simulink model "RTForwardVehicleSensorFusionTarget"  (R2024b)
settings: Solver=FixedStepAuto  StartTime=0.0  StopTime=Inf  RelTol=1e-3
PostLoadFcn:
  | helperSLForwardVehicleSensorFusionTargetSetup
undefined symbols (not defined in the file or in its folder): maxNumRadarDets, maxNumTracks, maxNumVisionDets, Ts
libraries: slrealtimeiplib x3, slrealtimeutilitieslib x3, simulink x2
CloseFcn:
  | helperSLForwardVehicleSensorFusionTargetCleanUp
settings Model: SimulationMode=external  Creator=The MathWorks, Inc.  LastModifiedBy=The MathWorks, Inc.
settings SolverCC: ConcurrentTasks=on  PositivePriorityOrder=on  MaxZcPerStep=1
settings DataIOCC: SignalLoggingName=rt_logsout
settings OptimizationCC: BlockReduction=off  OptimizeBlockIOStorage=off
settings DebuggingCC: TasksWithSamePriorityMsg=none  UnconnectedInputMsg=warning  UnconnectedOutputMsg=warning  UnconnectedLineMsg=warning  SubsystemReferenceDiagnosticForUnitTest=warning
settings HardwareCC: ProdBitPerLong=64  ProdLongLongMode=on  ProdHWDeviceType=Intel->x86-64 (Linux 64)
settings ModelReferenceCC: EnableRefExpFcnMdlSchedulingChecks=on
settings SFSimCC: SimTargetLang=C++
settings RTWCC: Description=Simulink Real-Time  SystemTargetFile=slrealtime.tlc  TemplateMakefile=slrealtime_default_tmf  Toolchain=Simulink Real-Time Toolchain  BuildConfiguration=Faster Runs  CodeExecutionProfiling=on  TargetLang=C++  GPUComputeCapability=3.5  DLArmComputeVersion=19.05
settings CodeAppCC: MaxIdLength=256
settings SimulinkRealTimeTargetCC: InstructionSetFMA=off  LogToMDFFile=off

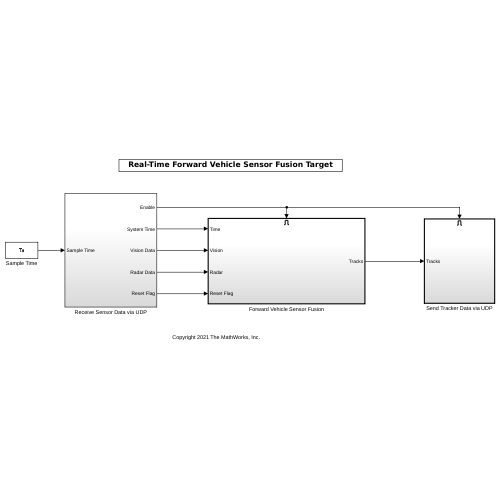
[thumbnail: Simulink's stored preview of the top-level diagram]
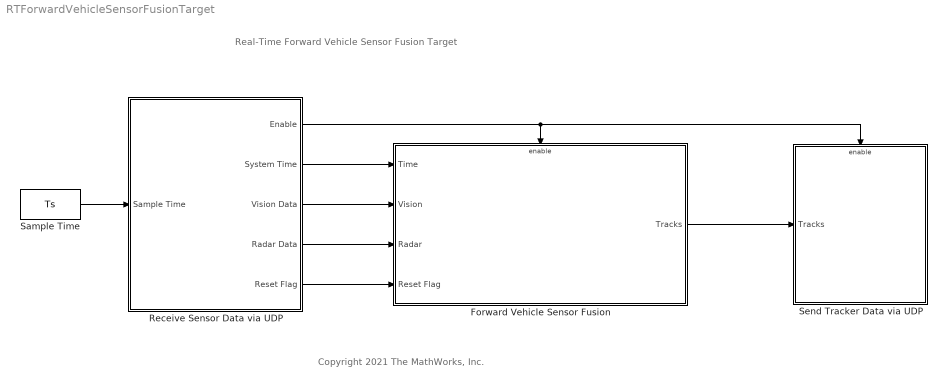
== system RTForwardVehicleSensorFusionTarget ==
  note: Real-Time Forward Vehicle Sensor Fusion Target
  note: Copyright 2021 The MathWorks, Inc.
  Forward Vehicle Sensor Fusion : Subsystem
  Receive Sensor Data via UDP : Subsystem
  Sample Time : Constant  Value=Ts  SampleTime=Ts
  Send Tracker Data via UDP : Subsystem
  wires:
  Sample Time/1 -> Receive Sensor Data via UDP/1(Sample Time)
  Receive Sensor Data via UDP/2(System Time) -> Forward Vehicle Sensor Fusion/1(Time)
  Receive Sensor Data via UDP/3(Vision Data) -> Forward Vehicle Sensor Fusion/2(Vision)
  Receive Sensor Data via UDP/4(Radar Data) -> Forward Vehicle Sensor Fusion/3(Radar)
  Receive Sensor Data via UDP/1(Enable) -> Forward Vehicle Sensor Fusion/Enable, Send Tracker Data via UDP/Enable
  Forward Vehicle Sensor Fusion/1(Tracks) -> Send Tracker Data via UDP/1(Tracks)
  Receive Sensor Data via UDP/5(Reset Flag) -> Forward Vehicle Sensor Fusion/4(Reset Flag)

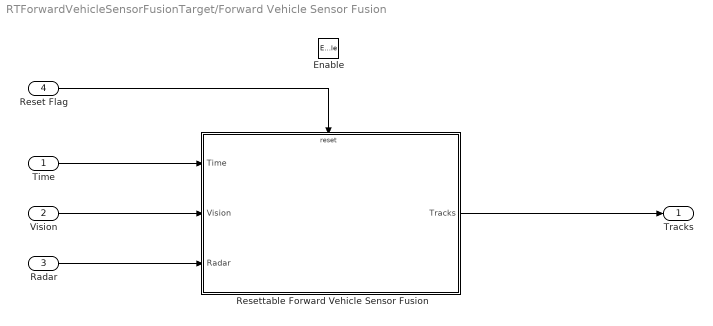
== system RTForwardVehicleSensorFusionTarget/Forward Vehicle Sensor Fusion ==
  Time : Inport
  Vision : Inport  Port=2  OutDataTypeStr=Bus: BusVision
  Radar : Inport  Port=3  OutDataTypeStr=Bus: BusRadar
  Reset Flag : Inport  Port=4
  Enable : EnablePort
  Resettable Forward Vehicle Sensor Fusion : Subsystem  TreatAsAtomicUnit=on
  Tracks : Outport
  wires:
  Time/1 -> Resettable Forward Vehicle Sensor Fusion/1(Time)
  Vision/1 -> Resettable Forward Vehicle Sensor Fusion/2(Vision)
  Radar/1 -> Resettable Forward Vehicle Sensor Fusion/3(Radar)
  Resettable Forward Vehicle Sensor Fusion/1(Tracks) -> Tracks/1
  Reset Flag/1 -> Resettable Forward Vehicle Sensor Fusion/Reset

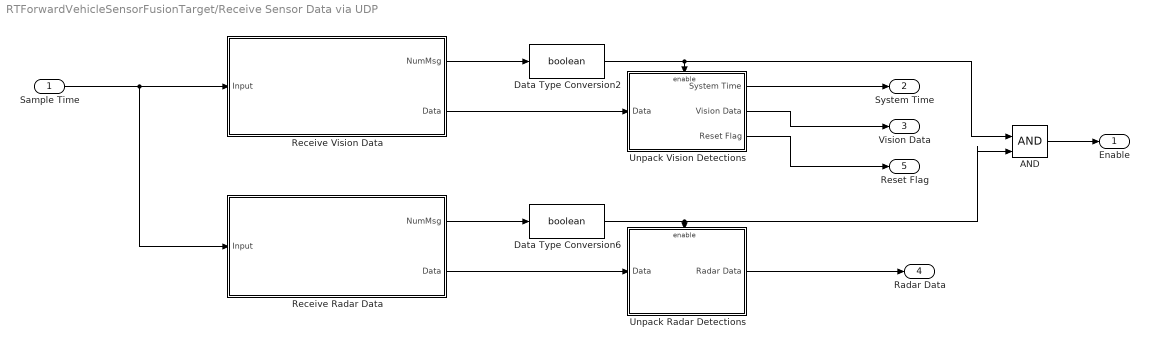
== system RTForwardVehicleSensorFusionTarget/Receive Sensor Data via UDP ==
  Sample Time : Inport
  AND : Logic  IconShape=distinctive  AllPortsSameDT=off  OutDataTypeStr=boolean
  Data Type Conversion2 : DataTypeConversion  OutDataTypeStr=boolean  SaturateOnIntegerOverflow=off  RndMeth=Floor
  Data Type Conversion6 : DataTypeConversion  OutDataTypeStr=boolean  SaturateOnIntegerOverflow=off  RndMeth=Floor
  Receive Radar Data : Subsystem
  Receive Vision Data : Subsystem
  Unpack Radar Detections : Subsystem
  Unpack Vision Detections : Subsystem
  Enable : Outport
  System Time : Outport  Port=2
  Vision Data : Outport  Port=3  OutDataTypeStr=Bus: BusVision
  Radar Data : Outport  Port=4  OutDataTypeStr=Bus: BusRadar
  Reset Flag : Outport  Port=5
  wires:
  Receive Vision Data/1(NumMsg) -> Data Type Conversion2/1
  Data Type Conversion2/1 -> AND/1, Unpack Vision Detections/Enable
  Receive Vision Data/2(Data) -> Unpack Vision Detections/1(Data)
  Unpack Vision Detections/1(System Time) -> System Time/1
  Unpack Radar Detections/1(Radar Data) -> Radar Data/1
  Receive Radar Data/2(Data) -> Unpack Radar Detections/1(Data)
  Receive Radar Data/1(NumMsg) -> Data Type Conversion6/1
  Data Type Conversion6/1 -> Unpack Radar Detections/Enable, AND/2
  Sample Time/1 -> Receive Radar Data/1(Input), Receive Vision Data/1(Input)
  Unpack Vision Detections/2(Vision Data) -> Vision Data/1
  AND/1 -> Enable/1
  Unpack Vision Detections/3(Reset Flag) -> Reset Flag/1

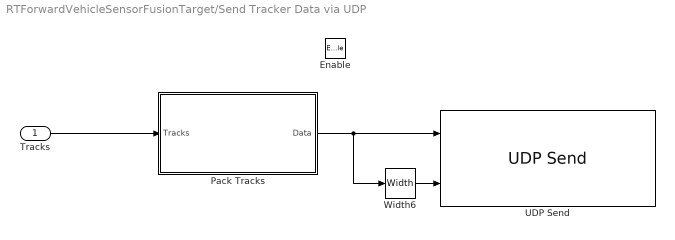
== system RTForwardVehicleSensorFusionTarget/Send Tracker Data via UDP ==
  Tracks : Inport
  Enable : EnablePort
  Pack Tracks : Subsystem
  UDP Send : slrealtimeiplib/UDP Send  useHostTargetConn=on  toAddress=10.1.10.16  toPort=8021  sampleTime=-1  enableMessage=off  ipAddress=10.1.10.17  localPort=-1
  Width6 : Width
  wires:
  Pack Tracks/1(Data) -> Width6/1, UDP Send/1
  Width6/1 -> UDP Send/2
  Tracks/1 -> Pack Tracks/1(Tracks)

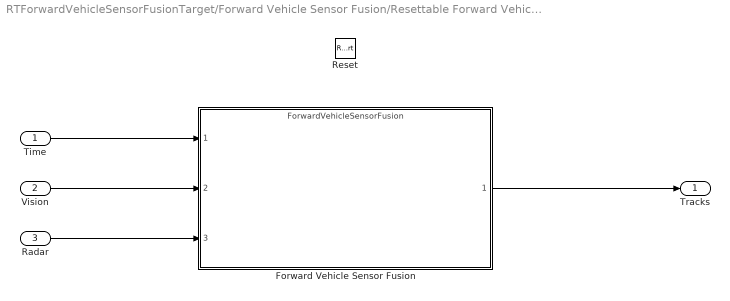
== system RTForwardVehicleSensorFusionTarget/Forward Vehicle Sensor Fusion/Resettable Forward Vehicle Sensor Fusion ==
  Time : Inport
  Vision : Inport  Port=2  OutDataTypeStr=Bus: BusVision
  Radar : Inport  Port=3  OutDataTypeStr=Bus: BusRadar
  Reset : ResetPort  DisableCoverage=on
  Forward Vehicle Sensor Fusion : ModelReference  ModelNameDialog=ForwardVehicleSensorFusion.slx  SimulationMode=Normal  CodeInterface=Top model  ModelReferenceVersion=10.0
  Tracks : Outport
  wires:
  Forward Vehicle Sensor Fusion/1 -> Tracks/1
  Time/1 -> Forward Vehicle Sensor Fusion/1
  Vision/1 -> Forward Vehicle Sensor Fusion/2
  Radar/1 -> Forward Vehicle Sensor Fusion/3

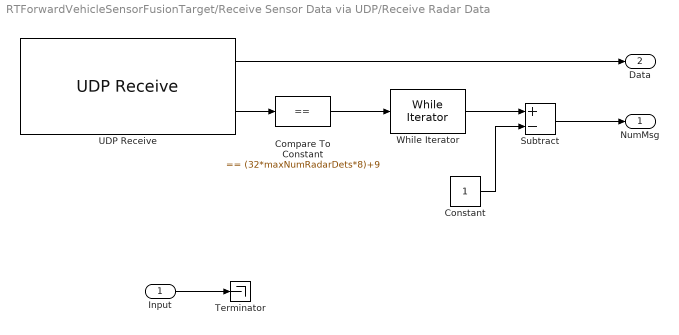
== system RTForwardVehicleSensorFusionTarget/Receive Sensor Data via UDP/Receive Radar Data ==
  Input : Inport
  Compare To Constant : simulink/Logic and Bit Operations/Compare To Constant  relop===  const=(32*maxNumRadarDets*8)+9  OutDataTypeStr=boolean
  Constant : Constant
  Subtract : Sum  Inputs=+-
  Terminator : Terminator
  UDP Receive : slrealtimeiplib/UDP Receive  useHostTargetConn=on  ipAddress=10.1.10.17  localPort=8002  rcvWidth=(32*maxNumRadarDets*8)+9  rcvFmAny=off  fmAddress=10.1.10.16  sampleTime=-1  enableMessage=off  maxPackets=1
  While Iterator : WhileIterator  WhileBlockType=do-while  ResetStates=reset  ShowIterationPort=on
  NumMsg : Outport
  Data : Outport  Port=2
  wires:
  Input/1 -> Terminator/1
  UDP Receive/2 -> Compare To Constant/1
  Subtract/1 -> NumMsg/1
  UDP Receive/1 -> Data/1
  Compare To Constant/1 -> While Iterator/1
  Constant/1 -> Subtract/2
  While Iterator/1 -> Subtract/1

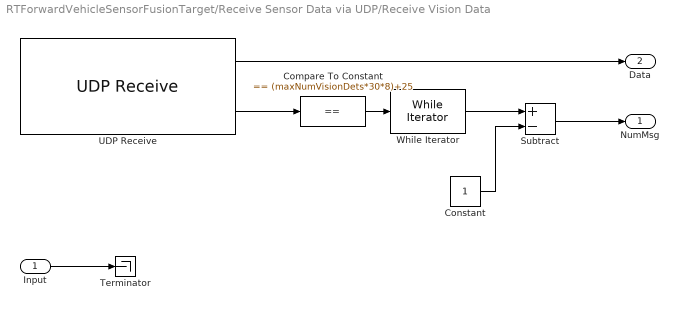
== system RTForwardVehicleSensorFusionTarget/Receive Sensor Data via UDP/Receive Vision Data ==
  Input : Inport
  Compare To Constant : simulink/Logic and Bit Operations/Compare To Constant  relop===  const=(maxNumVisionDets*30*8)+25  OutDataTypeStr=boolean
  Constant : Constant
  Subtract : Sum  Inputs=+-
  Terminator : Terminator
  UDP Receive : slrealtimeiplib/UDP Receive  useHostTargetConn=on  ipAddress=10.1.10.17  localPort=8001  rcvWidth=(maxNumVisionDets*30*8)+25  rcvFmAny=off  fmAddress=10.1.10.16  sampleTime=-1  enableMessage=off  maxPackets=1
  While Iterator : WhileIterator  WhileBlockType=do-while  ResetStates=reset  ShowIterationPort=on
  NumMsg : Outport
  Data : Outport  Port=2
  wires:
  Input/1 -> Terminator/1
  Compare To Constant/1 -> While Iterator/1
  UDP Receive/1 -> Data/1
  Constant/1 -> Subtract/2
  Subtract/1 -> NumMsg/1
  UDP Receive/2 -> Compare To Constant/1
  While Iterator/1 -> Subtract/1

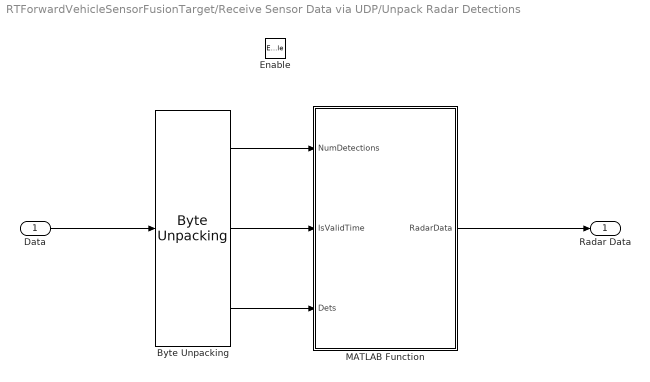
== system RTForwardVehicleSensorFusionTarget/Receive Sensor Data via UDP/Unpack Radar Detections ==
  Data : Inport
  Enable : EnablePort
  "Byte Unpacking " : slrealtimeutilitieslib/Byte Unpacking  MaskUnpackedDataTypes={'double', 'boolean', ['double']}  MaskUnpackedDataSizes={1,1,32*maxNumRadarDets}  MaskAlignment=1
  MATLAB Function : MATLAB Function  TreatAsAtomicUnit=on  mask{structObj=Simulink.Bus.createMATLABStruct('BusRadar');, maxNumDets=maxNumRadarDets}
      mask prompts: structObj "Output struct"
  Radar Data : Outport
  wires:
  "Byte Unpacking "/3 -> MATLAB Function/3(Dets)
  "Byte Unpacking "/2 -> MATLAB Function/2(IsValidTime)
  "Byte Unpacking "/1 -> MATLAB Function/1(NumDetections)
  Data/1 -> "Byte Unpacking "/1
  MATLAB Function/1(RadarData) -> Radar Data/1

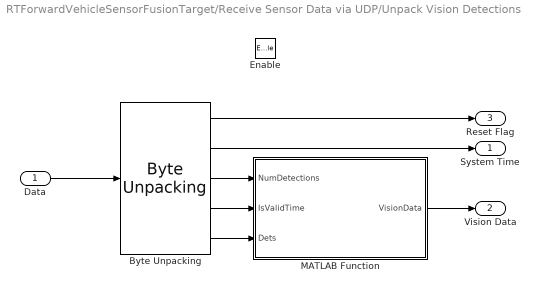
== system RTForwardVehicleSensorFusionTarget/Receive Sensor Data via UDP/Unpack Vision Detections ==
  Data : Inport
  Enable : EnablePort
  "Byte Unpacking " : slrealtimeutilitieslib/Byte Unpacking  MaskUnpackedDataTypes={'double','double','double', 'boolean', ['double']}  MaskUnpackedDataSizes={1,1,1,1,30*maxNumVisionDets}  MaskAlignment=1
  MATLAB Function : MATLAB Function  TreatAsAtomicUnit=on  mask{structObj=Simulink.Bus.createMATLABStruct('BusVision');, maxNumDets=maxNumVisionDets}
      mask prompts: structObj "Output struct"
  System Time : Outport
  Vision Data : Outport  Port=2
  Reset Flag : Outport  Port=3
  wires:
  Data/1 -> "Byte Unpacking "/1
  "Byte Unpacking "/2 -> System Time/1
  "Byte Unpacking "/3 -> MATLAB Function/1(NumDetections)
  "Byte Unpacking "/4 -> MATLAB Function/2(IsValidTime)
  "Byte Unpacking "/5 -> MATLAB Function/3(Dets)
  MATLAB Function/1(VisionData) -> Vision Data/1
  "Byte Unpacking "/1 -> Reset Flag/1

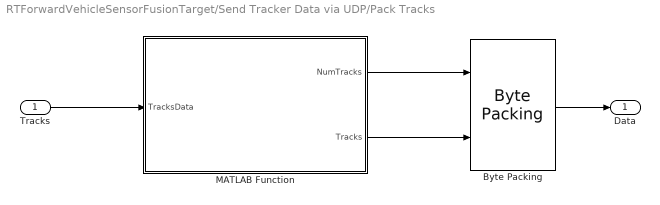
== system RTForwardVehicleSensorFusionTarget/Send Tracker Data via UDP/Pack Tracks ==
  Tracks : Inport
  Byte Packing : slrealtimeutilitieslib/Byte Packing  MaskPackedDataType=uint8  MaskUnpackedDataTypes={'double', ['double']}  MaskAlignment=1
  MATLAB Function : MATLAB Function  TreatAsAtomicUnit=on  mask{maxNumTracks=maxNumTracks}
  Data : Outport
  wires:
  Tracks/1 -> MATLAB Function/1(TracksData)
  Byte Packing/1 -> Data/1
  MATLAB Function/2(Tracks) -> Byte Packing/2
  MATLAB Function/1(NumTracks) -> Byte Packing/1

== matlab function RTForwardVehicleSensorFusionTarget/Send Tracker Data via UDP/Pack Tracks/MATLAB Function ==
  data: NumTracks output; Tracks output; TracksData input Bus: BusTrackerJPDA; maxNumTracks parameter
function [NumTracks, Tracks]  = busTrackerJPDAToUdpData(TracksData,...
                                                        maxNumTracks)
% busTrackerJPDAToUdpData function convert the tracks data structure
% (BusTrackerJPDA) into UDP data.

% Define data vector to store tracker data.
Tracks = zeros(1, maxNumTracks*61, 'double');

% Assign number of tracks to the output variable.
NumTracks = TracksData.NumTracks;

% Get sizes of structure elements into a vector.
sizesVector = [numel(TracksData.Tracks(1).TrackID),...
    numel(TracksData.Tracks(1).BranchID),...
    numel(TracksData.Tracks(1).SourceIndex),...
    numel(TracksData.Tracks(1).UpdateTime),...
    numel(TracksData.Tracks(1).Age),...
    numel(TracksData.Tracks(1).State),...
    numel(TracksData.Tracks(1).StateCovariance),...
    numel(TracksData.Tracks(1).ObjectClassID),...
    numel(TracksData.Tracks(1).TrackLogic),...
    numel(TracksData.Tracks(1).TrackLogicState),...
    numel(TracksData.Tracks(1).IsConfirmed),...
    numel(TracksData.Tracks(1).IsCoasted),...
    numel(TracksData.Tracks(1).IsSelfReported),...
    numel(TracksData.Tracks(1).ObjectAttributes(1).TargetIndex),...
    numel(TracksData.Tracks(1).ObjectAttributes(1).SNR),...
    numel(TracksData.Tracks(1).ObjectAttributes(2).TargetIndex),...
    numel(TracksData.Tracks(1).ObjectAttributes(2).SNR)];

% Assign tracker data to data vector.
k = 1;
for i=1:NumTracks
    Tracks(k) = TracksData.Tracks(i).TrackID;k=k+sizesVector(1);
    Tracks(k) = TracksData.Tracks(i).BranchID;k=k+sizesVector(2);
    Tracks(k) = TracksData.Tracks(i).SourceIndex;k=k+sizesVector(3);
    Tracks(k) = TracksData.Tracks(i).UpdateTime;k=k+sizesVector(4);
    Tracks(k) = TracksData.Tracks(i).Age;k=k+sizesVector(5);
    Tracks(k:k+sizesVector(6)-1) = TracksData.Tracks(i).State;k=k+sizesVector(6);
    Tracks(k:k+sizesVector(7)-1) = TracksData.Tracks(i).StateCovariance(:);k=k+sizesVector(7);
    Tracks(k) = TracksData.Tracks(i).ObjectClassID;k=k+sizesVector(8);
    Tracks(k) = TracksData.Tracks(i).TrackLogic;k=k+sizesVector(9);
    Tracks(k:k+sizesVector(10)-1) = TracksData.Tracks(i).TrackLogicState(:);k=k+sizesVector(10);
    Tracks(k) = TracksData.Tracks(i).IsConfirmed;k=k+sizesVector(11);
    Tracks(k) = TracksData.Tracks(i).IsCoasted;k=k+sizesVector(12);
    Tracks(k) = TracksData.Tracks(i).IsSelfReported;k=k+sizesVector(13);
    Tracks(k) = TracksData.Tracks(i).ObjectAttributes(1).TargetIndex;k=k+sizesVector(14);
    Tracks(k) = TracksData.Tracks(i).ObjectAttributes(1).SNR;k=k+sizesVector(15);
    Tracks(k) = TracksData.Tracks(i).ObjectAttributes(2).TargetIndex;k=k+sizesVector(16);
    Tracks(k) = TracksData.Tracks(i).ObjectAttributes(2).SNR;k=k+sizesVector(17);
end

end

== matlab function RTForwardVehicleSensorFusionTarget/Receive Sensor Data via UDP/Unpack Radar Detections/MATLAB Function ==
  data: NumDetections input; RadarData output Bus: BusRadar; IsValidTime input; Dets input; structObj parameter; maxNumDets parameter
function RadarData = udpDataToBusRadar(NumDetections, IsValidTime, Dets, ...
                                     structObj, maxNumDets)
% udpDataToBusRadar function fill up the radar detections structure
% (BusRadar) with received UDP data.

% Assign radar detections structure object to the output variable.
RadarData = structObj;

% Fill up the structure object with UDP data.
if NumDetections > maxNumDets
    RadarData.NumDetections = maxNumDets;
else
    RadarData.NumDetections = NumDetections;
end
RadarData.IsValidTime = IsValidTime;

% Get sizes of structure elements into a vector.
sizesVector = [numel(RadarData.Detections(1).Time), ...
               numel(RadarData.Detections(1).Measurement), ...
               numel(RadarData.Detections(1).MeasurementNoise(:)), ...
               numel(RadarData.Detections(1).SensorIndex), ...
               numel(RadarData.Detections(1).ObjectClassID), ...
               numel(RadarData.Detections(1).MeasurementParameters.Frame), ...
               numel(RadarData.Detections(1).MeasurementParameters.OriginPosition), ...
               numel(RadarData.Detections(1).MeasurementParameters.Orientation), ...
               numel(RadarData.Detections(1).MeasurementParameters.HasVelocity), ...
               numel(RadarData.Detections(1).MeasurementParameters.HasElevation), ...
               numel(RadarData.Detections(1).ObjectAttributes.TargetIndex), ...
               numel(RadarData.Detections(1).ObjectAttributes.SNR)];

% Fill up the structure object with UDP data.
k = 1;
for i=1:maxNumDets
    RadarData.Detections(i).Time = Dets(k);k=k+sizesVector(1);
    RadarData.Detections(i).Measurement = Dets(k:k+2);k=k+sizesVector(2);
    RadarData.Detections(i).MeasurementNoise(:) = Dets(k:k+sizesVector(3)-1);k=k+sizesVector(3);
    RadarData.Detections(i).SensorIndex = Dets(k);k=k+sizesVector(4);
    RadarData.Detections(i).ObjectClassID = Dets(k);k=k+sizesVector(5);
    RadarData.Detections(i).MeasurementParameters.Frame = drivingCoordinateFrameType(Dets(k));k=k+sizesVector(6);
    RadarData.Detections(i).MeasurementParameters.OriginPosition = Dets(k:k+2);k=k+sizesVector(7);
    RadarData.Detections(i).MeasurementParameters.Orientation = reshape(Dets(k:k+sizesVector(8)-1), [3 3]);k=k+sizesVector(8);
    RadarData.Detections(i).MeasurementParameters.HasVelocity = boolean(Dets(k));k=k+sizesVector(9);
    RadarData.Detections(i).MeasurementParameters.HasElevation = boolean(Dets(k));k=k+sizesVector(10);
    RadarData.Detections(i).ObjectAttributes.TargetIndex = Dets(k);k=k+sizesVector(11);
    RadarData.Detections(i).ObjectAttributes.SNR = Dets(k);k=k+sizesVector(12);
end

== matlab function RTForwardVehicleSensorFusionTarget/Receive Sensor Data via UDP/Unpack Vision Detections/MATLAB Function ==
  data: NumDetections input; VisionData output Bus: BusVision; IsValidTime input; Dets input; structObj parameter; maxNumDets parameter
function VisionData = udpDataToBusVision(NumDetections, IsValidTime, Dets, ...
                                       structObj, maxNumDets)
% udpDataToBusVision function fill up the vision detections structure
% (BusVision) with received UDP data.

% Assign vision detections structure object to the output variable.
VisionData = structObj;

% Fill up the structure object with UDP data.
if NumDetections > maxNumDets
    VisionData.NumDetections = maxNumDets;
else
    VisionData.NumDetections = NumDetections;
end
VisionData.IsValidTime = IsValidTime;

% Get sizes of structure elements into a vector.
sizesVector = [numel(VisionData.Detections(1).Time), ...
               numel(VisionData.Detections(1).Measurement), ...
               numel(VisionData.Detections(1).MeasurementNoise), ...
               numel(VisionData.Detections(1).SensorIndex), ...
               numel(VisionData.Detections(1).ObjectClassID), ...
               numel(VisionData.Detections(1).MeasurementParameters.Frame), ...
               numel(VisionData.Detections(1).MeasurementParameters.OriginPosition), ...
               numel(VisionData.Detections(1).MeasurementParameters.Orientation), ...
               numel(VisionData.Detections(1).MeasurementParameters.HasVelocity), ...
               numel(VisionData.Detections(1).ObjectAttributes.TargetIndex)];

% Fill up the structure object with UDP data.
k = 1;
for i=1:maxNumDets
    VisionData.Detections(i).Time = Dets(k);k=k+sizesVector(1);
    VisionData.Detections(i).Measurement = Dets(k:k+2);k=k+sizesVector(2);
    VisionData.Detections(i).MeasurementNoise(:) = Dets(k:k+sizesVector(3)-1);k=k+sizesVector(3);
    VisionData.Detections(i).SensorIndex = Dets(k);k=k+sizesVector(4);
    VisionData.Detections(i).ObjectClassID = Dets(k);k=k+sizesVector(5);
    VisionData.Detections(i).MeasurementParameters.Frame = drivingCoordinateFrameType(Dets(k));k=k+sizesVector(6);
    VisionData.Detections(i).MeasurementParameters.OriginPosition = Dets(k:k+2);k=k+sizesVector(7);
    VisionData.Detections(i).MeasurementParameters.Orientation = reshape(Dets(k:k+sizesVector(8)-1), [3 3]);k=k+sizesVector(8);
    VisionData.Detections(i).MeasurementParameters.HasVelocity = boolean(Dets(k));k=k+sizesVector(9);
    VisionData.Detections(i).ObjectAttributes.TargetIndex = Dets(k);k=k+sizesVector(10);
end
